simulink model "Halleys_Comet"  (R2018a)
settings: Solver=FixedStepAuto  StartTime=0.0  StopTime=T  FixedStep=10000  RelTol=1e-3
values from neighbouring files (symbols this model uses):
  a = -mu/(2*xi)    [AA279A_ECI2OE.m]    (also in AA279A_HW2.m = rp/(1-e(ii)); ECI2OE.m = inf; Halleys_Comet_Call.m = 2667966400; ISS_Call.m = 6781.5)
  e = norm(e_vec)    [AA279A_ECI2OE.m]    (also in AA279A_HW2.m = [0.7 0.0 1.9 1.0]; ECI2OE.m = norm(eVec); Halleys_Comet_Call.m = 0.967; ISS_Call.m = 0.0006483)
  M0 = 0    [Halleys_Comet_Call.m]    (also in ISS_Call.m = 0.9101; Iridium18_Call.m = 0.475253155318; Molniya331_Call.m = E - e*sin(E))
  n = [-h(2);h(1);0]    [AA279A_ECI2OE.m]    (also in AA279A_OE2ECI.m = sqrt(mu/a^3); ECI2OE.m = norm(nVec); Halleys_Comet_Call.m = sqrt(mu/(a^3)); ISS_Call.m = sqrt(mu/(a^3)))
settings Model: Creator=Marquito  LastModifiedBy=Marquito

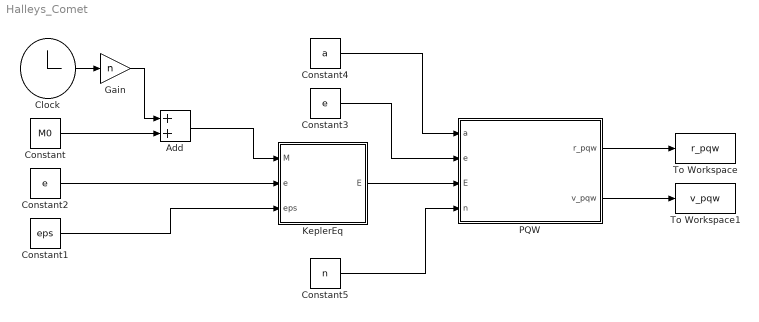
== system Halleys_Comet ==
  Add : Sum
  Clock : Clock
  Constant : Constant  Value=M0
  Constant1 : Constant  Value=eps
  Constant2 : Constant  Value=e
  Constant3 : Constant  Value=e
  Constant4 : Constant  Value=a
  Constant5 : Constant  Value=n
  Gain : Gain  Gain=n
  KeplerEq : MATLAB Function  TreatAsAtomicUnit=on
  PQW : MATLAB Function  TreatAsAtomicUnit=on
  To Workspace : ToWorkspace  VariableName=r_pqw  SampleTime=-1
  To Workspace1 : ToWorkspace  VariableName=v_pqw  SampleTime=-1
  wires:
  Clock/1 -> Gain/1
  Add/1 -> KeplerEq/1(M)
  KeplerEq/1(E) -> PQW/3(E)
  PQW/1(r_pqw) -> To Workspace/1
  PQW/2(v_pqw) -> To Workspace1/1
  Constant/1 -> Add/2
  Gain/1 -> Add/1
  Constant2/1 -> KeplerEq/2(e)
  Constant1/1 -> KeplerEq/3(eps)
  Constant3/1 -> PQW/2(e)
  Constant4/1 -> PQW/1(a)
  Constant5/1 -> PQW/4(n)

== matlab function Halleys_Comet/PQW ==
  data: a input; r_pqw output; e input; E input; v_pqw output; n input
function [r_pqw, v_pqw] = PQW(a, e, E, n)
% Compute Radius and Velocity of Orbit in Perifocal Coordinates
r_pqw = [a*(cos(E) - e); a*sqrt(1 - e^2)*sin(E); 0];
v_pqw = (a*n)/(1 - e*cos(E))*[-sin(E); sqrt(1 - e^2)*cos(E); 0];
end

== matlab function Halleys_Comet/KeplerEq ==
  data: M input; E output; e input; eps input
function E = KeplerEq(M,e,eps)
% Function solves Kepler's equation M = E-e*sin(E)
% Input - Mean Anomaly M [rad], Eccentricity e, and Epsilon 
% Output - Eccentric anomaly E [rad] 
En  = M;
Ens = En - (En-e*sin(En)- M)/(1 - e*cos(En));
while ( abs(Ens-En) > eps )
	En = Ens;
	Ens = En - (En - e*sin(En) - M)/(1 - e*cos(En));
end
E = Ens;
